simulink model "Pendulum_2_sim"  (R2018b)
settings: Solver=FixedStepAuto  StartTime=0.0  StopTime=5  FixedStep=0.002  RelTol=1e-3  EnableMultiTasking=on
libraries: simulink_extras x4, cstblocks x1, simulink x1
settings Model: ExtModeTrigDuration=10000  Creator=ACSI-MLC  LastModifiedBy=Brad
settings SolverCC: PositivePriorityOrder=on
settings RTWCC: Description=QUARC Win64 Target  SystemTargetFile=quarc_win64.tlc  TemplateMakefile=quarc_default_tmf
settings STFCustomTargetCC: TargetPreCompLibLocation=C:\PROGRA~3\QUARC\lib\2018b\win64\release  TargetLangStandard=C99 (ISO)  ConcurrentExecutionCompliant=on  GRTInterface=on  SystemTargetFile=quarc_win64.tlc
settings GRTTargetCC: TargetPreCompLibLocation=C:\PROGRA~3\QUARC\lib\2018b\win64\release  ParMdlRefBuildCompliant=off  CompOptLevelCompliant=off  CombineOutputUpdateFcns=off  MatFileLogging=off  CPPClassGenCompliant=off  GRTInterface=on  UseToolchainInfoCompliant=off  ExtMode=on  ExtModeMexFile=quarc_comm

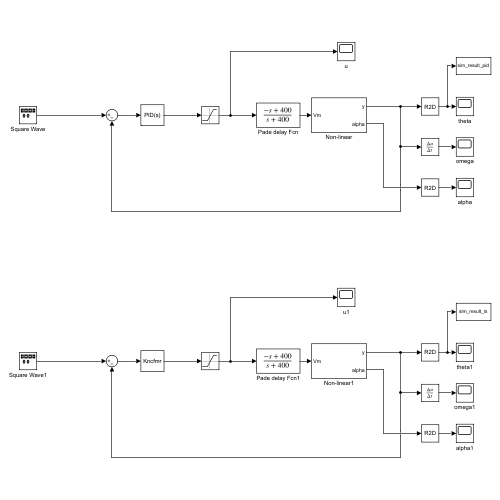
[thumbnail: Simulink's stored preview of the top-level diagram]
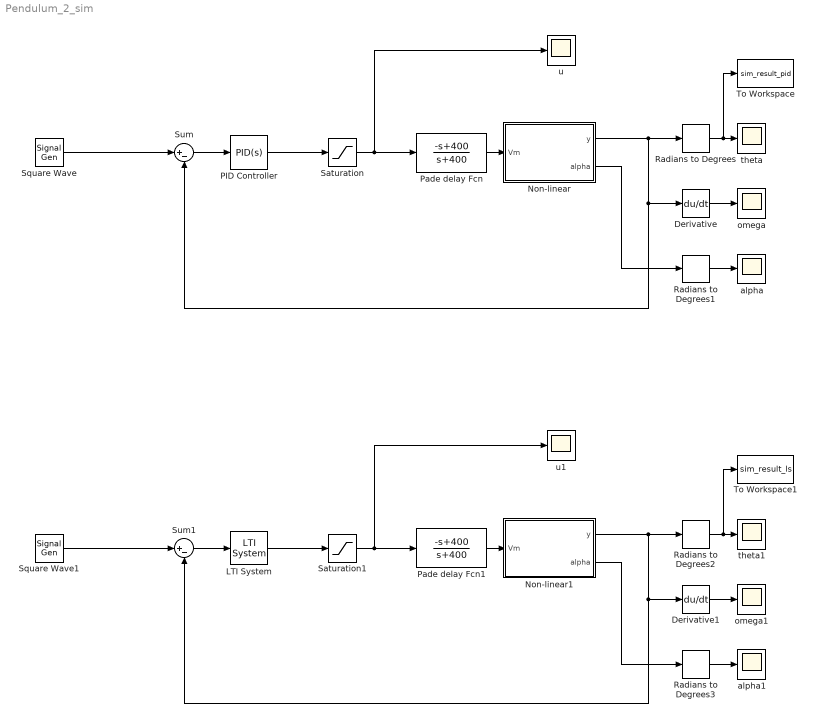
== system Pendulum_2_sim ==
  Derivative : Derivative
  Derivative1 : Derivative
  LTI System : cstblocks/LTI System  sys=Kncfmr  IC=[]
  Non-linear : Subsystem
  Non-linear1 : Subsystem
  PID Controller : simulink/Continuous/PID Controller  Controller=PID  Form=Parallel  TimeDomain=Continuous-time  SampleTime=-1  IntegratorMethod=Forward Euler  FilterMethod=Forward Euler  ControllerParametersSource=internal  P=48.1095208745377  I=132.090849888146  D=1.72349214314498  UseFilter=on  N=524.485779051163  TunerSelectOption=Transfer Function Based (PID Tuner App)  InitialConditionSource=internal  InitialConditionForIntegrator=0  InitialConditionForFilter=0  DifferentiatorICPrevScaledInput=0  ExternalReset=none  TrackingMode=off  Kt=1  LimitOutput=off  UpperSaturationLimit=10  LowerSaturationLimit=-10  LinearizeAsGain=on  AntiWindupMode=none  Kb=1  POutMin=[]  POutMax=[]  IOutMin=[]  IOutMax=[]  DOutMin=[]  DOutMax=[]  NOutMin=[]  NOutMax=[]  SumOutMin=[]  SumOutMax=[]  SaturationOutMin=[]  SaturationOutMax=[]  PParamMin=[]  PParamMax=[]  IParamMin=[]  IParamMax=[]  DParamMin=[]  DParamMax=[]  NParamMin=[]  NParamMax=[]  KbParamMin=[]  KbParamMax=[]  KtParamMin=[]  KtParamMax=[]  KbOutMin=[]  KbOutMax=[]  KtOutMin=[]  KtOutMax=[]  IntegratorOutMin=[]  IntegratorOutMax=[]  FilterOutMin=[]  FilterOutMax=[]  SumI1OutMin=[]  SumI1OutMax=[]  SumI2OutMin=[]  SumI2OutMax=[]  SumI3OutMin=[]  SumI3OutMax=[]  SumI4OutMin=[]  SumI4OutMax=[]  SumDOutMin=[]  SumDOutMax=[]  DifferentiatorOutMin=[]  DifferentiatorOutMax=[]  FilterDiffOutCoefMin=[]  FilterDiffOutCoefMax=[]  ReciprocalOutMin=[]  ReciprocalOutMax=[]  SumDenOutMin=[]  SumDenOutMax=[]  SumNumOutMin=[]  SumNumOutMax=[]  DivideOutMin=[]  DivideOutMax=[]  IntegratorContinuousStateAttributes=''  IntegratorStateMustResolveToSignalObject=off  IntegratorRTWStateStorageClass=Auto  FilterContinuousStateAttributes=''  FilterStateMustResolveToSignalObject=off  FilterRTWStateStorageClass=Auto  ParallelPVariant=InternalParameters  IdealPVariant=Disabled  IVariant=InternalParameters  DVariant=InternalParameters  IntegratorVariant=Continuous  SatVariant=Disabled  AWVariant=Passthrough  PCopyVariant=Disabled  TRVariant=Disabled  FdbkBlocksVariant=Forward  IdealPFdbkVariant=Disabled  SatFdbkVariant=Disabled  DerivativeFilterVariant=ContFilter  NVariant=InternalParameters  NCopyVariant=Disabled  FilterICVariant=InternalICsFilter  IntegratorICVariant=InternalICs  ExternalResetVariant=Disabled  TRSumVariant=Passthrough  SumFdbkVariant=Disabled  SumVariant=Sum_PID
  Pade delay Fcn : TransferFcn  Numerator=[-1 400]  Denominator=[1 400]
  Pade delay Fcn1 : TransferFcn  Numerator=[-1 400]  Denominator=[1 400]
  Radians to Degrees{,1..3} (4 alike) : simulink_extras/Transformations/Radians to Degrees
  Saturation : Saturate  UpperLimit=10  LowerLimit=-10
  Saturation1 : Saturate  UpperLimit=10  LowerLimit=-10
  Square Wave : SignalGenerator  WaveForm=square  Amplitude=deg2rad(10)  Frequency=0.5
  Square Wave1 : SignalGenerator  WaveForm=square  Amplitude=deg2rad(10)  Frequency=0.5
  Sum : Sum  Inputs=|+-
  Sum1 : Sum  Inputs=|+-
  To Workspace : ToWorkspace  VariableName=sim_result_pid  SampleTime=-1
  To Workspace1 : ToWorkspace  VariableName=sim_result_ls  SampleTime=-1
  alpha : Scope
  alpha1 : Scope
  omega : Scope
  omega1 : Scope
  theta : Scope
  theta1 : Scope
  u : Scope
  u1 : Scope
  wires:
  Radians to Degrees/1 -> To Workspace/1, theta/1
  Derivative/1 -> omega/1
  PID Controller/1 -> Saturation/1
  Non-linear/1(y) -> Sum/2, Derivative/1, Radians to Degrees/1
  Sum/1 -> PID Controller/1
  Square Wave/1 -> Sum/1
  Saturation/1 -> Pade delay Fcn/1, u/1
  Radians to Degrees1/1 -> alpha/1
  Pade delay Fcn/1 -> Non-linear/1(Vm)
  Non-linear/2(alpha) -> Radians to Degrees1/1
  Pade delay Fcn1/1 -> Non-linear1/1(Vm)
  Non-linear1/2(alpha) -> Radians to Degrees3/1
  LTI System/1 -> Saturation1/1
  Non-linear1/1(y) -> Sum1/2, Derivative1/1, Radians to Degrees2/1
  Saturation1/1 -> Pade delay Fcn1/1, u1/1
  Radians to Degrees2/1 -> To Workspace1/1, theta1/1
  Derivative1/1 -> omega1/1
  Square Wave1/1 -> Sum1/1
  Sum1/1 -> LTI System/1
  Radians to Degrees3/1 -> alpha1/1

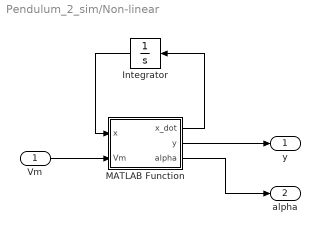
== system Pendulum_2_sim/Non-linear ==
  Vm : Inport
  Integrator : Integrator  InitialCondition=[0 0 0 0]
  MATLAB Function : MATLAB Function  TreatAsAtomicUnit=on
  y : Outport
  alpha : Outport  Port=2
  wires:
  MATLAB Function/1(x_dot) -> Integrator/1
  MATLAB Function/2(y) -> y/1
  Integrator/1 -> MATLAB Function/1(x)
  Vm/1 -> MATLAB Function/2(Vm)
  MATLAB Function/3(alpha) -> alpha/1

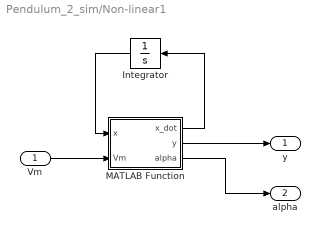
== system Pendulum_2_sim/Non-linear1 ==
  Vm : Inport
  Integrator : Integrator  InitialCondition=[0 0 0 0]
  MATLAB Function : MATLAB Function  TreatAsAtomicUnit=on
  y : Outport
  alpha : Outport  Port=2
  wires:
  MATLAB Function/1(x_dot) -> Integrator/1
  MATLAB Function/2(y) -> y/1
  Integrator/1 -> MATLAB Function/1(x)
  Vm/1 -> MATLAB Function/2(Vm)
  MATLAB Function/3(alpha) -> alpha/1

== matlab function Pendulum_2_sim/Non-linear1/MATLAB Function ==
  data: x input; x_dot output; Vm input; y output; alpha output
function [x_dot, y, alpha] = fcn(x, Vm)
x_dot = [x(2); get_theta_ddot(x(1),x(2),x(3),x(4),Vm); x(4); get_alpha_ddot(x(1),x(2),x(3),x(4),Vm)];
y = x(1);
alpha = x(3);
end

== matlab function Pendulum_2_sim/Non-linear/MATLAB Function ==
  data: x input; x_dot output; Vm input; y output; alpha output
function [x_dot, y, alpha] = fcn(x, Vm)
x_dot = [x(2); get_theta_ddot(x(1),x(2),x(3),x(4),Vm); x(4); get_alpha_ddot(x(1),x(2),x(3),x(4),Vm)];
y = x(1);
alpha = x(3);
end
